simulink model "simulink_model_parteA"  (R2023b)
settings: Solver=VariableStepAuto  StartTime=0.0  StopTime=400  RelTol=1e-3
libraries: fuzblock x1
settings Model: Creator=jbsantos  LastModifiedBy=jbsantos

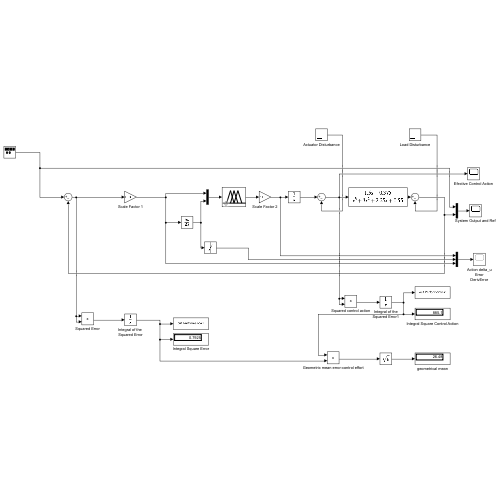
[thumbnail: Simulink's stored preview of the top-level diagram]
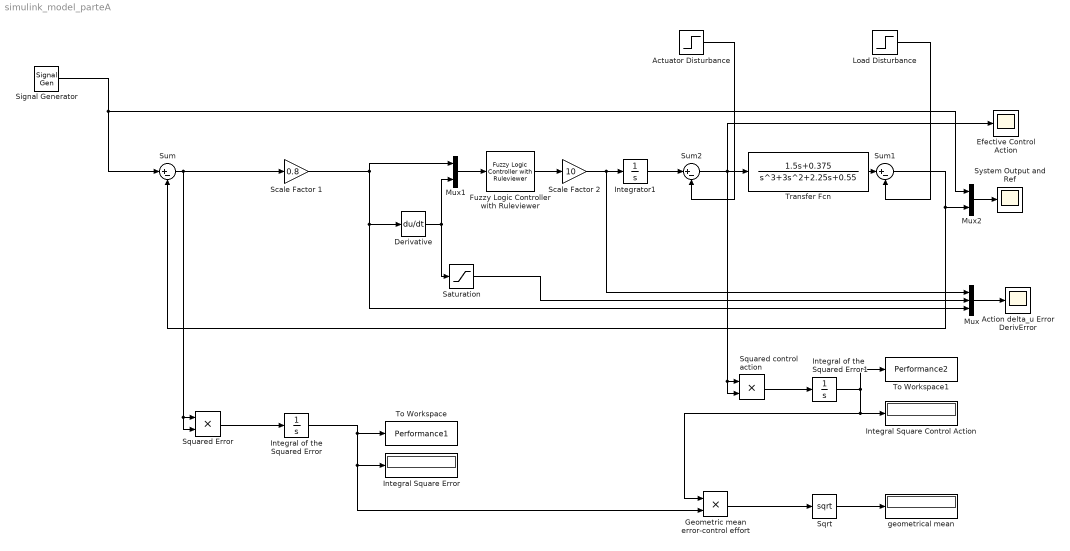
== system simulink_model_parteA ==
  Action delta_u Error DerivError : Scope
  Actuator Disturbance : Step  Time=200  SampleTime=0
  Derivative : Derivative
  Efective Control Action : Scope
  Fuzzy Logic Controller with Ruleviewer : fuzblock/Fuzzy Logic  Controller  with Ruleviewer  fismatrix=sugeno25_gauss  Ts=1
  Geometric mean error-control effort : Product
  Integral Square Control Action : Display
  Integral Square Error : Display
  Integral of the Squared Error1 : Integrator
  Integral of the Squared Error : Integrator
  Integrator1 : Integrator
  Load Disturbance : Step  Time=300  SampleTime=0
  Mux : Mux  Inputs=3
  Mux1 : Mux  Inputs=2
  Mux2 : Mux  Inputs=2
  Saturation : Saturate
  Scale Factor 1 : Gain  Gain=0.8
  Scale Factor 2 : Gain  Gain=10
  Signal Generator : SignalGenerator  Frequency=0.02  Units=rad/sec
  Sqrt : Sqrt
  Squared Error : Product
  Squared control action : Product
  Sum : Sum  Inputs=|+-
  Sum1 : Sum  Inputs=|+-
  Sum2 : Sum  Inputs=|+-
  System Output and Ref : Scope
  To Workspace : ToWorkspace  VariableName=Performance1  SaveFormat=Timeseries  SampleTime=-1
  To Workspace1 : ToWorkspace  VariableName=Performance2  SaveFormat=Timeseries  SampleTime=-1
  Transfer Fcn : TransferFcn  Numerator=[1.5 0.375]  Denominator=[1 3 2.25 0.55]
  geometrical mean : Display
  wires:
  Signal Generator/1 -> Sum/1, Mux2/1
  Sum/1 -> Squared Error/2, Squared Error/1, Scale Factor 1/1
  Squared Error/1 -> Integral of the Squared Error/1
  Integral of the Squared Error/1 -> Integral Square Error/1, Geometric mean error-control effort/2, To Workspace/1
  Scale Factor 1/1 -> Mux1/1, Derivative/1, Mux/3
  Derivative/1 -> Saturation/1, Mux1/2
  Transfer Fcn/1 -> Sum1/1
  Sum1/1 -> Sum/2, Mux2/2
  Load Disturbance/1 -> Sum1/2
  Mux2/1 -> System Output and Ref/1
  Saturation/1 -> Mux/2
  Scale Factor 2/1 -> Integrator1/1, Mux/1
  Integrator1/1 -> Sum2/1
  Sum2/1 -> Efective Control Action/1, Transfer Fcn/1, Squared control action/2, Squared control action/1
  Actuator Disturbance/1 -> Sum2/2
  Squared control action/1 -> Integral of the Squared Error1/1
  Integral of the Squared Error1/1 -> Geometric mean error-control effort/1, Integral Square Control Action/1, To Workspace1/1
  Mux/1 -> Action delta_u Error DerivError/1
  Geometric mean error-control effort/1 -> Sqrt/1
  Sqrt/1 -> geometrical mean/1
  Mux1/1 -> Fuzzy Logic Controller with Ruleviewer/1
  Fuzzy Logic Controller with Ruleviewer/1 -> Scale Factor 2/1
